simulink library "powerlib_extras"  (Simulink 6.0)
settings: Solver=ode45  SolverMode=SingleTasking  StartTime=0.0  StopTime=10.0  RelTol=1e-3
values from neighbouring files (symbols this model uses):
  Ts = get(handles.edit1,'string')    [powergui.m]
undefined symbols (not defined in the file or in its folder): Ac, Bc, Cc, Dc, Delay_discrete, dend, DiscIntNeverNeededParam, extra_sc, j, numd, test_alpha
libraries: powerlib2 x112, powerlib_extras x70, simulink_extras x25, simulink x12, powerlib_models x8
(part 9 of 9)

== system powerlib_extras/Discrete  Control Blocks/Discrete Synchronized 12-Pulse Generator/12 Flip-Flops/6 Flip-Flop1 ==
  S : Inport  Port=1  LatchInput=off
  R : Inport  Port=2  LatchInput=off
  Demux : Demux  Outputs=6
  Demux1 : Demux  Outputs=6
  Mux : Mux  Inputs=6
  S-R Flip-Flop1 : Subsystem  mask(SRFlipFlop){initial_condition=0, Ts=Ts}
      mask prompts: initial_condition "Initial condition:"; Ts "Sample time:"
      mask help: S-R Flip Flop Block
  S-R Flip-Flop2 : Subsystem  mask(SRFlipFlop){initial_condition=0, Ts=Ts}
      mask prompts: initial_condition "Initial condition:"; Ts "Sample time:"
      mask help: S-R Flip Flop Block
  S-R Flip-Flop3 : Subsystem  mask(SRFlipFlop){initial_condition=0, Ts=Ts}
      mask prompts: initial_condition "Initial condition:"; Ts "Sample time:"
      mask help: S-R Flip Flop Block
  S-R Flip-Flop4 : Subsystem  mask(SRFlipFlop){initial_condition=0, Ts=Ts}
      mask prompts: initial_condition "Initial condition:"; Ts "Sample time:"
      mask help: S-R Flip Flop Block
  S-R Flip-Flop5 : Subsystem  mask(SRFlipFlop){initial_condition=0, Ts=Ts}
      mask prompts: initial_condition "Initial condition:"; Ts "Sample time:"
      mask help: S-R Flip Flop Block
  S-R Flip-Flop6 : Subsystem  mask(SRFlipFlop){initial_condition=0, Ts=Ts}
      mask prompts: initial_condition "Initial condition:"; Ts "Sample time:"
      mask help: S-R Flip Flop Block
  Terminator{,1..5} (6 alike) : Terminator
  Q : Outport
  wires:
  Demux1/6 -> S-R Flip-Flop6/2(R)
  Demux1/5 -> S-R Flip-Flop5/2(R)
  Demux1/4 -> S-R Flip-Flop4/2(R)
  Demux1/3 -> S-R Flip-Flop3/2(R)
  Demux1/2 -> S-R Flip-Flop2/2(R)
  Demux1/1 -> S-R Flip-Flop1/2(R)
  R/1 -> Demux1/1
  Demux/5 -> S-R Flip-Flop5/1(S)
  Demux/6 -> S-R Flip-Flop6/1(S)
  S/1 -> Demux/1
  Demux/4 -> S-R Flip-Flop4/1(S)
  Demux/3 -> S-R Flip-Flop3/1(S)
  Demux/2 -> S-R Flip-Flop2/1(S)
  Demux/1 -> S-R Flip-Flop1/1(S)
  S-R Flip-Flop1/2(!Q) -> Terminator/1
  S-R Flip-Flop6/1(Q) -> Mux/6
  Mux/1 -> Q/1
  S-R Flip-Flop5/1(Q) -> Mux/5
  S-R Flip-Flop4/1(Q) -> Mux/4
  S-R Flip-Flop3/1(Q) -> Mux/3
  S-R Flip-Flop2/1(Q) -> Mux/2
  S-R Flip-Flop1/1(Q) -> Mux/1
  S-R Flip-Flop2/2(!Q) -> Terminator1/1
  S-R Flip-Flop3/2(!Q) -> Terminator2/1
  S-R Flip-Flop4/2(!Q) -> Terminator3/1
  S-R Flip-Flop5/2(!Q) -> Terminator4/1
  S-R Flip-Flop6/2(!Q) -> Terminator5/1

== system powerlib_extras/Discrete  Control Blocks/Discrete Synchronized 6-Pulse Generator/6 Flip-Flop/S-R Flip-Flop1 ==
  S : Inport  Port=1  LatchInput=off
  R : Inport  Port=2  LatchInput=off
  Demux : Demux  Outputs=2
  Logic : CombinatorialLogic  TruthTable=[0 1;0 1;1 0;0 1;1 0;0 1;1 0;1 0]
  Mux : Mux  Inputs=3
  Unit Delay : UnitDelay  Orientation=left  X0=initial_condition  SampleTime=Ts
  Q : Outport  InitialOutput=0
  !Q : Outport  Port=2  InitialOutput=1
  wires:
  Mux/1 -> Logic/1
  Logic/1 -> Demux/1
  Demux/2 -> !Q/1
  Demux/1 -> Q/1, Unit Delay/1
  Unit Delay/1 -> Mux/1
  S/1 -> Mux/2
  R/1 -> Mux/3

== system powerlib_extras/Discrete  Control Blocks/Discrete Synchronized 6-Pulse Generator/6 Flip-Flop/S-R Flip-Flop2 ==
  S : Inport  Port=1  LatchInput=off
  R : Inport  Port=2  LatchInput=off
  Demux : Demux  Outputs=2
  Logic : CombinatorialLogic  TruthTable=[0 1;0 1;1 0;0 1;1 0;0 1;1 0;1 0]
  Mux : Mux  Inputs=3
  Unit Delay : UnitDelay  Orientation=left  X0=initial_condition  SampleTime=Ts
  Q : Outport  InitialOutput=0
  !Q : Outport  Port=2  InitialOutput=1
  wires:
  R/1 -> Mux/3
  S/1 -> Mux/2
  Unit Delay/1 -> Mux/1
  Demux/1 -> Unit Delay/1, Q/1
  Demux/2 -> !Q/1
  Logic/1 -> Demux/1
  Mux/1 -> Logic/1

== system powerlib_extras/Discrete  Control Blocks/Discrete Synchronized 6-Pulse Generator/6 Flip-Flop/S-R Flip-Flop3 ==
  S : Inport  Port=1  LatchInput=off
  R : Inport  Port=2  LatchInput=off
  Demux : Demux  Outputs=2
  Logic : CombinatorialLogic  TruthTable=[0 1;0 1;1 0;0 1;1 0;0 1;1 0;1 0]
  Mux : Mux  Inputs=3
  Unit Delay : UnitDelay  Orientation=left  X0=initial_condition  SampleTime=Ts
  Q : Outport  InitialOutput=0
  !Q : Outport  Port=2  InitialOutput=1
  wires:
  Mux/1 -> Logic/1
  Logic/1 -> Demux/1
  Demux/2 -> !Q/1
  Demux/1 -> Q/1, Unit Delay/1
  Unit Delay/1 -> Mux/1
  S/1 -> Mux/2
  R/1 -> Mux/3

== system powerlib_extras/Discrete  Control Blocks/Discrete Synchronized 6-Pulse Generator/6 Flip-Flop/S-R Flip-Flop4 ==
  S : Inport  Port=1  LatchInput=off
  R : Inport  Port=2  LatchInput=off
  Demux : Demux  Outputs=2
  Logic : CombinatorialLogic  TruthTable=[0 1;0 1;1 0;0 1;1 0;0 1;1 0;1 0]
  Mux : Mux  Inputs=3
  Unit Delay : UnitDelay  Orientation=left  X0=initial_condition  SampleTime=Ts
  Q : Outport  InitialOutput=0
  !Q : Outport  Port=2  InitialOutput=1
  wires:
  R/1 -> Mux/3
  S/1 -> Mux/2
  Unit Delay/1 -> Mux/1
  Demux/1 -> Unit Delay/1, Q/1
  Demux/2 -> !Q/1
  Logic/1 -> Demux/1
  Mux/1 -> Logic/1

== system powerlib_extras/Discrete  Control Blocks/Discrete Synchronized 6-Pulse Generator/6 Flip-Flop/S-R Flip-Flop5 ==
  S : Inport  Port=1  LatchInput=off
  R : Inport  Port=2  LatchInput=off
  Demux : Demux  Outputs=2
  Logic : CombinatorialLogic  TruthTable=[0 1;0 1;1 0;0 1;1 0;0 1;1 0;1 0]
  Mux : Mux  Inputs=3
  Unit Delay : UnitDelay  Orientation=left  X0=initial_condition  SampleTime=Ts
  Q : Outport  InitialOutput=0
  !Q : Outport  Port=2  InitialOutput=1
  wires:
  Mux/1 -> Logic/1
  Logic/1 -> Demux/1
  Demux/2 -> !Q/1
  Demux/1 -> Q/1, Unit Delay/1
  Unit Delay/1 -> Mux/1
  S/1 -> Mux/2
  R/1 -> Mux/3

== system powerlib_extras/Discrete  Control Blocks/Discrete Synchronized 6-Pulse Generator/6 Flip-Flop/S-R Flip-Flop6 ==
  S : Inport  Port=1  LatchInput=off
  R : Inport  Port=2  LatchInput=off
  Demux : Demux  Outputs=2
  Logic : CombinatorialLogic  TruthTable=[0 1;0 1;1 0;0 1;1 0;0 1;1 0;1 0]
  Mux : Mux  Inputs=3
  Unit Delay : UnitDelay  Orientation=left  X0=initial_condition  SampleTime=Ts
  Q : Outport  InitialOutput=0
  !Q : Outport  Port=2  InitialOutput=1
  wires:
  R/1 -> Mux/3
  S/1 -> Mux/2
  Unit Delay/1 -> Mux/1
  Demux/1 -> Unit Delay/1, Q/1
  Demux/2 -> !Q/1
  Logic/1 -> Demux/1
  Mux/1 -> Logic/1

== system powerlib_extras/Discrete  Control Blocks/Discrete 12-Pulse HVDC Control /Functions (Discrete)/Current Regulator/Kp Linearisation ==
  note: Kp Linearization
  note: Silvano Casoria
      | Laboratoire simulation de reseaux, IREQ
  Alpha_lin : Inport  Port=1  LatchInput=off
  Kp : Inport  Port=2  LatchInput=off
  Inv : Inport  Port=3  LatchInput=off
  Min_lin : Inport  Port=4  LatchInput=off
  Max_lin : Inport  Port=5  LatchInput=off
  Constant3 : Constant  Value=On_lin
  Data Type  Conversion : DataTypeConversion  OutDataTypeMode=boolean  SaturateOnIntegerOverflow=on  RndMeth=Zero
  Logical Operator : Logic  Operator=NOT
  Logical Operator1 : Logic  Operator=NOT
  Math Function : Math  Operator=reciprocal  SaturateOnIntegerOverflow=on
  Prod2 : Product  Inputs=3  SaturateOnIntegerOverflow=on  InputSameDT=on
  S6 : Subsystem
      mask Type: Limiter with External Limits
      mask Display: disp('      Limiter\n')
  Switch : Switch  Threshold=0.5  SaturateOnIntegerOverflow=on  InputSameDT=on
  Switch1 : Switch  Threshold=0.5  SaturateOnIntegerOverflow=on  InputSameDT=on
  Trigonometric Function : Trigonometry
  Trigonometric Function1 : Trigonometry
  k : Gain  Gain=pi/180  SaturateOnIntegerOverflow=on
  k1 : Gain  Gain=pi/180  SaturateOnIntegerOverflow=on
  Kp_lin : Outport  InitialOutput=0
  wires:
  Logical Operator1/1 -> Switch1/2  "Off"
  Prod2/1 -> Switch1/3
  Switch1/1 -> Kp_lin/1
  Switch/1 -> k1/1
  k1/1 -> Trigonometric Function/1
  S6/1("  ") -> k/1
  Trigonometric Function/1 -> Prod2/1
  Logical Operator/1 -> Switch/2
  Inv/1 -> Logical Operator/1
  Kp/1 -> Switch1/1, Prod2/3
  k/1 -> Trigonometric Function1/1
  Trigonometric Function1/1 -> Math Function/1
  Math Function/1 -> Prod2/2
  Alpha_lin/1 -> S6/2(In)
  Max_lin/1 -> Switch/3, S6/1(MAX)
  Min_lin/1 -> Switch/1, S6/3(MIN)
  Constant3/1 -> Data Type  Conversion/1
  Data Type  Conversion/1 -> Logical Operator1/1

== system powerlib_extras/Discrete  Control Blocks/Discrete 12-Pulse HVDC Control /Functions (Discrete)/Current Regulator/S16 ==
  note: Gain * dt
  note: INTEGRATOR with External limits & Reset & Hold
  Max : Inport  Port=1  LatchInput=off
  Min : Inport  Port=2  LatchInput=off
  In : Inport  Port=3  LatchInput=off
  Reset : Inport  Port=4  LatchInput=off
  Hold : Inport  Port=5  LatchInput=off
  Reset Value : Inport  Port=6  LatchInput=off
  Gain1 : Gain  Gain=k*st  SaturateOnIntegerOverflow=on
  IC = ic : UnitDelay  X0=ic  SampleTime=st
  Logical Operator4 : Logic  Operator=OR
  MinMax : MinMax  Inputs=2  SaturateOnIntegerOverflow=on  InputSameDT=on
  MinMax1 : MinMax  Function=max  Inputs=2  SaturateOnIntegerOverflow=on  InputSameDT=on
  S6 : Subsystem
      mask Type: Limiter with External Limits
      mask Display: disp('      Limiter\n')
  Sum : Sum  SaturateOnIntegerOverflow=on  InputSameDT=on
  Switch2 : Switch  Threshold=0.5  SaturateOnIntegerOverflow=on  InputSameDT=on
  Switch3 : Switch  Threshold=0.5  SaturateOnIntegerOverflow=on  InputSameDT=on
  Switch7 : Switch  Threshold=0.5  SaturateOnIntegerOverflow=on  InputSameDT=on
  Out : Outport  InitialOutput=0
  wires:
  Switch7/1 -> Switch3/1, Sum/2, Switch2/1
  IC = ic/1 -> Switch7/3
  Min/1 -> MinMax1/2, Switch3/3
  Switch3/1 -> MinMax1/1
  MinMax1/1 -> S6/3(MIN)
  MinMax/1 -> S6/1(MAX)
  Reset Value/1 -> Switch7/1
  Max/1 -> MinMax/2, Switch2/3
  Switch2/1 -> MinMax/1
  Logical Operator4/1 -> Switch3/2, Switch2/2
  Reset/1 -> Logical Operator4/2, Switch7/2
  Hold/1 -> Logical Operator4/1
  S6/1("  ") -> IC = ic/1, Out/1
  Sum/1 -> S6/2(In)
  In/1 -> Gain1/1
  Gain1/1 -> Sum/1

== system powerlib_extras/Discrete  Control Blocks/Discrete 12-Pulse HVDC Control /Functions (Discrete)/Current Regulator/S6 ==
  note: Limiter
      | with external
      | limits
  MAX : Inport  Port=1  LatchInput=off
  In : Inport  Port=2  LatchInput=off
  MIN : Inport  Port=3  LatchInput=off
  MinMax : MinMax  Function=max  Inputs=2  SaturateOnIntegerOverflow=on  InputSameDT=on
  MinMax1 : MinMax  Inputs=2  SaturateOnIntegerOverflow=on  InputSameDT=on
  "  " : Outport  InitialOutput=0
  wires:
  MinMax1/1 -> MinMax/2
  MAX/1 -> MinMax1/1
  MIN/1 -> MinMax/1
  MinMax/1 -> "  "/1
  In/1 -> MinMax1/2

== system powerlib_extras/Discrete  Control Blocks/Discrete 12-Pulse HVDC Control /Functions (Discrete)/VDCOL/PB_R ==
  note: LOW PASS Filter & RESET
      | (Zoh methode)
  note: Silvano Casoria
      | Laboratoire simulation de reseaux, IREQ
  "In " : Inport  Port=1  LatchInput=off
  Reset : Inport  Port=2  LatchInput=off
  T : Inport  Port=3  LatchInput=off
  Constant : Constant  Value=dt
  IC= ic : UnitDelay  Orientation=left  X0=ic  SampleTime=dt
  Math Function : Math  Operator=reciprocal  SaturateOnIntegerOverflow=on
  Product : Product  Inputs=3  SaturateOnIntegerOverflow=on  InputSameDT=on
  Sum : Sum  Inputs=+-  SaturateOnIntegerOverflow=on  InputSameDT=on
  Sum1 : Sum  SaturateOnIntegerOverflow=on  InputSameDT=on
  Switch : Switch  Threshold=0.5  SaturateOnIntegerOverflow=on  InputSameDT=on
  Out : Outport  InitialOutput=0
  wires:
  Constant/1 -> Product/3
  T/1 -> Math Function/1
  Math Function/1 -> Product/1
  Sum/1 -> Product/2
  Product/1 -> Sum1/1
  Switch/1 -> IC= ic/1
  Sum1/1 -> Switch/3, Out/1
  Reset/1 -> Switch/2
  "In "/1 -> Switch/1, Sum/1
  IC= ic/1 -> Sum1/2, Sum/2

== system powerlib_extras/Discrete  Control Blocks/Discrete 12-Pulse HVDC Control /Functions (Discrete)/Voltage Regulator/Kp Linearisation ==
  note: Kp Linearization
  Alpha_lin : Inport  Port=1  LatchInput=off
  Kp : Inport  Port=2  LatchInput=off
  Inv : Inport  Port=3  LatchInput=off
  Min_lin : Inport  Port=4  LatchInput=off
  Max_lin : Inport  Port=5  LatchInput=off
  Constant3 : Constant  Value=On_lin
  Data Type  Conversion : DataTypeConversion  OutDataTypeMode=boolean  SaturateOnIntegerOverflow=on  RndMeth=Zero
  Logical Operator : Logic  Operator=NOT
  Logical Operator1 : Logic  Operator=NOT
  Math Function : Math  Operator=reciprocal  SaturateOnIntegerOverflow=on
  Prod2 : Product  Inputs=3  SaturateOnIntegerOverflow=on  InputSameDT=on
  S6 : Subsystem
      mask Type: Limiter with External Limits
      mask Display: disp('      Limiter\n')
  Switch : Switch  Threshold=0.5  SaturateOnIntegerOverflow=on  InputSameDT=on
  Switch1 : Switch  Threshold=0.5  SaturateOnIntegerOverflow=on  InputSameDT=on
  Trigonometric Function : Trigonometry
  Trigonometric Function1 : Trigonometry
  k : Gain  Gain=pi/180  SaturateOnIntegerOverflow=on
  k1 : Gain  Gain=pi/180  SaturateOnIntegerOverflow=on
  Kp_lin : Outport  InitialOutput=0
  wires:
  Min_lin/1 -> S6/3(MIN), Switch/1
  Max_lin/1 -> S6/1(MAX), Switch/3
  Alpha_lin/1 -> S6/2(In)
  Math Function/1 -> Prod2/2
  Trigonometric Function1/1 -> Math Function/1
  k/1 -> Trigonometric Function1/1
  Kp/1 -> Prod2/3, Switch1/1
  Inv/1 -> Logical Operator/1
  Logical Operator/1 -> Switch/2
  Trigonometric Function/1 -> Prod2/1
  S6/1("  ") -> k/1
  k1/1 -> Trigonometric Function/1
  Switch/1 -> k1/1
  Switch1/1 -> Kp_lin/1
  Prod2/1 -> Switch1/3
  Logical Operator1/1 -> Switch1/2  "Off"
  Constant3/1 -> Data Type  Conversion/1
  Data Type  Conversion/1 -> Logical Operator1/1

== system powerlib_extras/Discrete  Control Blocks/Discrete 12-Pulse HVDC Control /Functions (Discrete)/Voltage Regulator/S16 ==
  note: INTEGRATOR with External limits & Reset & Hold
  note: Gain * dt
  Max : Inport  Port=1  LatchInput=off
  Min : Inport  Port=2  LatchInput=off
  In : Inport  Port=3  LatchInput=off
  Reset : Inport  Port=4  LatchInput=off
  Hold : Inport  Port=5  LatchInput=off
  Reset Value : Inport  Port=6  LatchInput=off
  Gain1 : Gain  Gain=k*st  SaturateOnIntegerOverflow=on
  IC = ic : UnitDelay  X0=ic  SampleTime=st
  Logical Operator4 : Logic  Operator=OR
  MinMax : MinMax  Inputs=2  SaturateOnIntegerOverflow=on  InputSameDT=on
  MinMax1 : MinMax  Function=max  Inputs=2  SaturateOnIntegerOverflow=on  InputSameDT=on
  S6 : Subsystem
      mask Type: Limiter with External Limits
      mask Display: disp('      Limiter\n')
  Sum : Sum  SaturateOnIntegerOverflow=on  InputSameDT=on
  Switch2 : Switch  Threshold=0.5  SaturateOnIntegerOverflow=on  InputSameDT=on
  Switch3 : Switch  Threshold=0.5  SaturateOnIntegerOverflow=on  InputSameDT=on
  Switch7 : Switch  Threshold=0.5  SaturateOnIntegerOverflow=on  InputSameDT=on
  Out : Outport  InitialOutput=0
  wires:
  Gain1/1 -> Sum/1
  In/1 -> Gain1/1
  Sum/1 -> S6/2(In)
  S6/1("  ") -> Out/1, IC = ic/1
  Hold/1 -> Logical Operator4/1
  Reset/1 -> Switch7/2, Logical Operator4/2
  Logical Operator4/1 -> Switch2/2, Switch3/2
  Switch2/1 -> MinMax/1
  Max/1 -> Switch2/3, MinMax/2
  Reset Value/1 -> Switch7/1
  MinMax/1 -> S6/1(MAX)
  MinMax1/1 -> S6/3(MIN)
  Switch3/1 -> MinMax1/1
  Min/1 -> Switch3/3, MinMax1/2
  IC = ic/1 -> Switch7/3
  Switch7/1 -> Switch2/1, Sum/2, Switch3/1

== system powerlib_extras/Discrete  Control Blocks/Discrete 12-Pulse HVDC Control /Functions (Discrete)/Voltage Regulator/S6 ==
  note: Limiter
      | with external
      | limits
  MAX : Inport  Port=1  LatchInput=off
  In : Inport  Port=2  LatchInput=off
  MIN : Inport  Port=3  LatchInput=off
  MinMax : MinMax  Function=max  Inputs=2  SaturateOnIntegerOverflow=on  InputSameDT=on
  MinMax1 : MinMax  Inputs=2  SaturateOnIntegerOverflow=on  InputSameDT=on
  "  " : Outport  InitialOutput=0
  wires:
  In/1 -> MinMax1/2
  MinMax/1 -> "  "/1
  MIN/1 -> MinMax/1
  MAX/1 -> MinMax1/1
  MinMax1/1 -> MinMax/2

== system powerlib_extras/Discrete  Control Blocks/Discrete HVDC Controller/Current Regulator/Kp Linearisation/S6 ==
  note: Limiter
      | with external
      | limits
  MAX : Inport  Port=1  LatchInput=off
  In : Inport  Port=2  LatchInput=off
  MIN : Inport  Port=3  LatchInput=off
  MinMax : MinMax  Function=max  Inputs=2  SaturateOnIntegerOverflow=on  InputSameDT=on
  MinMax1 : MinMax  Inputs=2  SaturateOnIntegerOverflow=on  InputSameDT=on
  "  " : Outport  InitialOutput=0
  wires:
  MinMax1/1 -> MinMax/2
  MAX/1 -> MinMax1/1
  MIN/1 -> MinMax/1
  MinMax/1 -> "  "/1
  In/1 -> MinMax1/2

== system powerlib_extras/Discrete  Control Blocks/Discrete HVDC Controller/Current Regulator/S16/S6 ==
  note: Limiter
      | with external
      | limits
  MAX : Inport  Port=1  LatchInput=off
  In : Inport  Port=2  LatchInput=off
  MIN : Inport  Port=3  LatchInput=off
  MinMax : MinMax  Function=max  Inputs=2  SaturateOnIntegerOverflow=on  InputSameDT=on
  MinMax1 : MinMax  Inputs=2  SaturateOnIntegerOverflow=on  InputSameDT=on
  "  " : Outport  InitialOutput=0
  wires:
  MinMax1/1 -> MinMax/2
  MAX/1 -> MinMax1/1
  MIN/1 -> MinMax/1
  MinMax/1 -> "  "/1
  In/1 -> MinMax1/2

== system powerlib_extras/Discrete  Control Blocks/Discrete HVDC Controller/Gamma Regulator/Gamma Regulator/Kp Linearisation ==
  note: Kp Linearization
  Alpha_lin : Inport  Port=1  LatchInput=off
  Kp : Inport  Port=2  LatchInput=off
  Inv : Inport  Port=3  LatchInput=off
  Min_lin : Inport  Port=4  LatchInput=off
  Max_lin : Inport  Port=5  LatchInput=off
  Constant3 : Constant  Value=On_lin
  Data Type  Conversion : DataTypeConversion  OutDataTypeMode=boolean  SaturateOnIntegerOverflow=on  RndMeth=Zero
  Logical Operator : Logic  Operator=NOT
  Logical Operator1 : Logic  Operator=NOT
  Math Function : Math  Operator=reciprocal  SaturateOnIntegerOverflow=on
  Prod2 : Product  Inputs=3  SaturateOnIntegerOverflow=on  InputSameDT=on
  S6 : Subsystem
      mask Type: Limiter with External Limits
      mask Display: disp('      Limiter\n')
  Switch : Switch  Threshold=0.5  SaturateOnIntegerOverflow=on  InputSameDT=on
  Switch1 : Switch  Threshold=0.5  SaturateOnIntegerOverflow=on  InputSameDT=on
  Trigonometric Function : Trigonometry
  Trigonometric Function1 : Trigonometry
  k : Gain  Gain=pi/180  SaturateOnIntegerOverflow=on
  k1 : Gain  Gain=pi/180  SaturateOnIntegerOverflow=on
  Kp_lin : Outport  InitialOutput=0
  wires:
  Data Type  Conversion/1 -> Logical Operator1/1
  Constant3/1 -> Data Type  Conversion/1
  Logical Operator1/1 -> Switch1/2  "Off"
  Prod2/1 -> Switch1/3
  Switch1/1 -> Kp_lin/1
  Switch/1 -> k1/1
  k1/1 -> Trigonometric Function/1
  S6/1("  ") -> k/1
  Trigonometric Function/1 -> Prod2/1
  Logical Operator/1 -> Switch/2
  Inv/1 -> Logical Operator/1
  Kp/1 -> Switch1/1, Prod2/3
  k/1 -> Trigonometric Function1/1
  Trigonometric Function1/1 -> Math Function/1
  Math Function/1 -> Prod2/2
  Alpha_lin/1 -> S6/2(In)
  Max_lin/1 -> Switch/3, S6/1(MAX)
  Min_lin/1 -> Switch/1, S6/3(MIN)

== system powerlib_extras/Discrete  Control Blocks/Discrete HVDC Controller/Gamma Regulator/Gamma Regulator/S16 ==
  note: Gain * dt
  note: INTEGRATOR with External limits & Reset & Hold
  Max : Inport  Port=1  LatchInput=off
  Min : Inport  Port=2  LatchInput=off
  In : Inport  Port=3  LatchInput=off
  Reset : Inport  Port=4  LatchInput=off
  Hold : Inport  Port=5  LatchInput=off
  Reset Value : Inport  Port=6  LatchInput=off
  Gain1 : Gain  Gain=k*st  SaturateOnIntegerOverflow=on
  IC = ic : UnitDelay  X0=ic  SampleTime=st
  Logical Operator4 : Logic  Operator=OR
  MinMax : MinMax  Inputs=2  SaturateOnIntegerOverflow=on  InputSameDT=on
  MinMax1 : MinMax  Function=max  Inputs=2  SaturateOnIntegerOverflow=on  InputSameDT=on
  S6 : Subsystem
      mask Type: Limiter with External Limits
      mask Display: disp('      Limiter\n')
  Sum : Sum  SaturateOnIntegerOverflow=on  InputSameDT=on
  Switch2 : Switch  Threshold=0.5  SaturateOnIntegerOverflow=on  InputSameDT=on
  Switch3 : Switch  Threshold=0.5  SaturateOnIntegerOverflow=on  InputSameDT=on
  Switch7 : Switch  Threshold=0.5  SaturateOnIntegerOverflow=on  InputSameDT=on
  Out : Outport  InitialOutput=0
  wires:
  Switch7/1 -> Switch3/1, Sum/2, Switch2/1
  IC = ic/1 -> Switch7/3
  Min/1 -> MinMax1/2, Switch3/3
  Switch3/1 -> MinMax1/1
  MinMax1/1 -> S6/3(MIN)
  MinMax/1 -> S6/1(MAX)
  Reset Value/1 -> Switch7/1
  Max/1 -> MinMax/2, Switch2/3
  Switch2/1 -> MinMax/1
  Logical Operator4/1 -> Switch3/2, Switch2/2
  Reset/1 -> Logical Operator4/2, Switch7/2
  Hold/1 -> Logical Operator4/1
  S6/1("  ") -> IC = ic/1, Out/1
  Sum/1 -> S6/2(In)
  In/1 -> Gain1/1
  Gain1/1 -> Sum/1

== system powerlib_extras/Discrete  Control Blocks/Discrete HVDC Controller/Gamma Regulator/Gamma Regulator/S6 ==
  note: Limiter
      | with external
      | limits
  MAX : Inport  Port=1  LatchInput=off
  In : Inport  Port=2  LatchInput=off
  MIN : Inport  Port=3  LatchInput=off
  MinMax : MinMax  Function=max  Inputs=2  SaturateOnIntegerOverflow=on  InputSameDT=on
  MinMax1 : MinMax  Inputs=2  SaturateOnIntegerOverflow=on  InputSameDT=on
  "  " : Outport  InitialOutput=0
  wires:
  MinMax1/1 -> MinMax/2
  MAX/1 -> MinMax1/1
  MIN/1 -> MinMax/1
  MinMax/1 -> "  "/1
  In/1 -> MinMax1/2

== system powerlib_extras/Discrete  Control Blocks/Discrete HVDC Controller/Voltage Regulator/Voltage Regulator/Kp Linearisation ==
  note: Kp Linearization
  Alpha_lin : Inport  Port=1  LatchInput=off
  Kp : Inport  Port=2  LatchInput=off
  Inv : Inport  Port=3  LatchInput=off
  Min_lin : Inport  Port=4  LatchInput=off
  Max_lin : Inport  Port=5  LatchInput=off
  Constant3 : Constant  Value=On_lin
  Data Type  Conversion : DataTypeConversion  OutDataTypeMode=boolean  SaturateOnIntegerOverflow=on  RndMeth=Zero
  Logical Operator : Logic  Operator=NOT
  Logical Operator1 : Logic  Operator=NOT
  Math Function : Math  Operator=reciprocal  SaturateOnIntegerOverflow=on
  Prod2 : Product  Inputs=3  SaturateOnIntegerOverflow=on  InputSameDT=on
  S6 : Subsystem
      mask Type: Limiter with External Limits
      mask Display: disp('      Limiter\n')
  Switch : Switch  Threshold=0.5  SaturateOnIntegerOverflow=on  InputSameDT=on
  Switch1 : Switch  Threshold=0.5  SaturateOnIntegerOverflow=on  InputSameDT=on
  Trigonometric Function : Trigonometry
  Trigonometric Function1 : Trigonometry
  k : Gain  Gain=pi/180  SaturateOnIntegerOverflow=on
  k1 : Gain  Gain=pi/180  SaturateOnIntegerOverflow=on
  Kp_lin : Outport  InitialOutput=0
  wires:
  Min_lin/1 -> S6/3(MIN), Switch/1
  Max_lin/1 -> S6/1(MAX), Switch/3
  Alpha_lin/1 -> S6/2(In)
  Math Function/1 -> Prod2/2
  Trigonometric Function1/1 -> Math Function/1
  k/1 -> Trigonometric Function1/1
  Kp/1 -> Prod2/3, Switch1/1
  Inv/1 -> Logical Operator/1
  Logical Operator/1 -> Switch/2
  Trigonometric Function/1 -> Prod2/1
  S6/1("  ") -> k/1
  k1/1 -> Trigonometric Function/1
  Switch/1 -> k1/1
  Switch1/1 -> Kp_lin/1
  Prod2/1 -> Switch1/3
  Logical Operator1/1 -> Switch1/2  "Off"
  Constant3/1 -> Data Type  Conversion/1
  Data Type  Conversion/1 -> Logical Operator1/1

== system powerlib_extras/Discrete  Control Blocks/Discrete HVDC Controller/Voltage Regulator/Voltage Regulator/S16 ==
  note: INTEGRATOR with External limits & Reset & Hold
  note: Gain * dt
  Max : Inport  Port=1  LatchInput=off
  Min : Inport  Port=2  LatchInput=off
  In : Inport  Port=3  LatchInput=off
  Reset : Inport  Port=4  LatchInput=off
  Hold : Inport  Port=5  LatchInput=off
  Reset Value : Inport  Port=6  LatchInput=off
  Gain1 : Gain  Gain=k*st  SaturateOnIntegerOverflow=on
  IC = ic : UnitDelay  X0=ic  SampleTime=st
  Logical Operator4 : Logic  Operator=OR
  MinMax : MinMax  Inputs=2  SaturateOnIntegerOverflow=on  InputSameDT=on
  MinMax1 : MinMax  Function=max  Inputs=2  SaturateOnIntegerOverflow=on  InputSameDT=on
  S6 : Subsystem
      mask Type: Limiter with External Limits
      mask Display: disp('      Limiter\n')
  Sum : Sum  SaturateOnIntegerOverflow=on  InputSameDT=on
  Switch2 : Switch  Threshold=0.5  SaturateOnIntegerOverflow=on  InputSameDT=on
  Switch3 : Switch  Threshold=0.5  SaturateOnIntegerOverflow=on  InputSameDT=on
  Switch7 : Switch  Threshold=0.5  SaturateOnIntegerOverflow=on  InputSameDT=on
  Out : Outport  InitialOutput=0
  wires:
  Gain1/1 -> Sum/1
  In/1 -> Gain1/1
  Sum/1 -> S6/2(In)
  S6/1("  ") -> Out/1, IC = ic/1
  Hold/1 -> Logical Operator4/1
  Reset/1 -> Switch7/2, Logical Operator4/2
  Logical Operator4/1 -> Switch2/2, Switch3/2
  Switch2/1 -> MinMax/1
  Max/1 -> Switch2/3, MinMax/2
  Reset Value/1 -> Switch7/1
  MinMax/1 -> S6/1(MAX)
  MinMax1/1 -> S6/3(MIN)
  Switch3/1 -> MinMax1/1
  Min/1 -> Switch3/3, MinMax1/2
  IC = ic/1 -> Switch7/3
  Switch7/1 -> Switch2/1, Sum/2, Switch3/1

== system powerlib_extras/Discrete  Control Blocks/Discrete HVDC Controller/Voltage Regulator/Voltage Regulator/S6 ==
  note: Limiter
      | with external
      | limits
  MAX : Inport  Port=1  LatchInput=off
  In : Inport  Port=2  LatchInput=off
  MIN : Inport  Port=3  LatchInput=off
  MinMax : MinMax  Function=max  Inputs=2  SaturateOnIntegerOverflow=on  InputSameDT=on
  MinMax1 : MinMax  Inputs=2  SaturateOnIntegerOverflow=on  InputSameDT=on
  "  " : Outport  InitialOutput=0
  wires:
  In/1 -> MinMax1/2
  MinMax/1 -> "  "/1
  MIN/1 -> MinMax/1
  MAX/1 -> MinMax1/1
  MinMax1/1 -> MinMax/2

== system powerlib_extras/Discrete  Control Blocks/Discrete SV PWM Generator/SV Modulator Pattern #1/Generate  pulse pattern/Determine interval of the PWM period based on Ta Tb and To ==
  TaTbTo : Inport  Port=1  LatchInput=off
  Constant7 : Constant
  Demux1 : Demux  Outputs=6
  Relational Operator{,1..5} (6 alike) : RelationalOperator
  Subsystem : Subsystem
  Sum1 : Sum  Inputs=+++++++  SaturateOnIntegerOverflow=on
  Triangle : simulink/Sources/Repeating Sequence  rep_seq_t=[0 1/Fc]  rep_seq_y=[0 1/Fc]
  Tn : Outport
  wires:
  TaTbTo/1 -> Subsystem/1(TaTbTo)
  Subsystem/1(Timing) -> Demux1/1
  Triangle/1 -> Relational Operator4/1, Relational Operator3/1, Relational Operator2/1, Relational Operator1/1, Relational Operator/1, Relational Operator5/1
  Relational Operator4/1 -> Sum1/7
  Relational Operator3/1 -> Sum1/6
  Relational Operator2/1 -> Sum1/5
  Relational Operator1/1 -> Sum1/4
  Relational Operator/1 -> Sum1/3
  Relational Operator5/1 -> Sum1/2
  Constant7/1 -> Sum1/1
  Demux1/1 -> Relational Operator5/2
  Demux1/2 -> Relational Operator/2
  Demux1/3 -> Relational Operator1/2
  Demux1/4 -> Relational Operator2/2
  Demux1/5 -> Relational Operator3/2
  Demux1/6 -> Relational Operator4/2
  Sum1/1 -> Tn/1

== system powerlib_extras/Discrete  Control Blocks/Discrete Synchronized 12-Pulse Generator/12 Flip-Flops/6 Flip-Flop/S-R Flip-Flop1 ==
  S : Inport  Port=1  LatchInput=off
  R : Inport  Port=2  LatchInput=off
  Demux : Demux  Outputs=2
  Logic : CombinatorialLogic  TruthTable=[0 1;0 1;1 0;0 1;1 0;0 1;1 0;1 0]
  Mux : Mux  Inputs=3
  Unit Delay : UnitDelay  Orientation=left  X0=initial_condition  SampleTime=Ts
  Q : Outport  InitialOutput=0
  !Q : Outport  Port=2  InitialOutput=1
  wires:
  R/1 -> Mux/3
  S/1 -> Mux/2
  Unit Delay/1 -> Mux/1
  Demux/1 -> Unit Delay/1, Q/1
  Demux/2 -> !Q/1
  Logic/1 -> Demux/1
  Mux/1 -> Logic/1

== system powerlib_extras/Discrete  Control Blocks/Discrete Synchronized 12-Pulse Generator/12 Flip-Flops/6 Flip-Flop/S-R Flip-Flop2 ==
  S : Inport  Port=1  LatchInput=off
  R : Inport  Port=2  LatchInput=off
  Demux : Demux  Outputs=2
  Logic : CombinatorialLogic  TruthTable=[0 1;0 1;1 0;0 1;1 0;0 1;1 0;1 0]
  Mux : Mux  Inputs=3
  Unit Delay : UnitDelay  Orientation=left  X0=initial_condition  SampleTime=Ts
  Q : Outport  InitialOutput=0
  !Q : Outport  Port=2  InitialOutput=1
  wires:
  Mux/1 -> Logic/1
  Logic/1 -> Demux/1
  Demux/2 -> !Q/1
  Demux/1 -> Q/1, Unit Delay/1
  Unit Delay/1 -> Mux/1
  S/1 -> Mux/2
  R/1 -> Mux/3

== system powerlib_extras/Discrete  Control Blocks/Discrete Synchronized 12-Pulse Generator/12 Flip-Flops/6 Flip-Flop/S-R Flip-Flop3 ==
  S : Inport  Port=1  LatchInput=off
  R : Inport  Port=2  LatchInput=off
  Demux : Demux  Outputs=2
  Logic : CombinatorialLogic  TruthTable=[0 1;0 1;1 0;0 1;1 0;0 1;1 0;1 0]
  Mux : Mux  Inputs=3
  Unit Delay : UnitDelay  Orientation=left  X0=initial_condition  SampleTime=Ts
  Q : Outport  InitialOutput=0
  !Q : Outport  Port=2  InitialOutput=1
  wires:
  R/1 -> Mux/3
  S/1 -> Mux/2
  Unit Delay/1 -> Mux/1
  Demux/1 -> Unit Delay/1, Q/1
  Demux/2 -> !Q/1
  Logic/1 -> Demux/1
  Mux/1 -> Logic/1

== system powerlib_extras/Discrete  Control Blocks/Discrete Synchronized 12-Pulse Generator/12 Flip-Flops/6 Flip-Flop/S-R Flip-Flop4 ==
  S : Inport  Port=1  LatchInput=off
  R : Inport  Port=2  LatchInput=off
  Demux : Demux  Outputs=2
  Logic : CombinatorialLogic  TruthTable=[0 1;0 1;1 0;0 1;1 0;0 1;1 0;1 0]
  Mux : Mux  Inputs=3
  Unit Delay : UnitDelay  Orientation=left  X0=initial_condition  SampleTime=Ts
  Q : Outport  InitialOutput=0
  !Q : Outport  Port=2  InitialOutput=1
  wires:
  Mux/1 -> Logic/1
  Logic/1 -> Demux/1
  Demux/2 -> !Q/1
  Demux/1 -> Q/1, Unit Delay/1
  Unit Delay/1 -> Mux/1
  S/1 -> Mux/2
  R/1 -> Mux/3

== system powerlib_extras/Discrete  Control Blocks/Discrete Synchronized 12-Pulse Generator/12 Flip-Flops/6 Flip-Flop/S-R Flip-Flop5 ==
  S : Inport  Port=1  LatchInput=off
  R : Inport  Port=2  LatchInput=off
  Demux : Demux  Outputs=2
  Logic : CombinatorialLogic  TruthTable=[0 1;0 1;1 0;0 1;1 0;0 1;1 0;1 0]
  Mux : Mux  Inputs=3
  Unit Delay : UnitDelay  Orientation=left  X0=initial_condition  SampleTime=Ts
  Q : Outport  InitialOutput=0
  !Q : Outport  Port=2  InitialOutput=1
  wires:
  R/1 -> Mux/3
  S/1 -> Mux/2
  Unit Delay/1 -> Mux/1
  Demux/1 -> Unit Delay/1, Q/1
  Demux/2 -> !Q/1
  Logic/1 -> Demux/1
  Mux/1 -> Logic/1

== system powerlib_extras/Discrete  Control Blocks/Discrete Synchronized 12-Pulse Generator/12 Flip-Flops/6 Flip-Flop/S-R Flip-Flop6 ==
  S : Inport  Port=1  LatchInput=off
  R : Inport  Port=2  LatchInput=off
  Demux : Demux  Outputs=2
  Logic : CombinatorialLogic  TruthTable=[0 1;0 1;1 0;0 1;1 0;0 1;1 0;1 0]
  Mux : Mux  Inputs=3
  Unit Delay : UnitDelay  Orientation=left  X0=initial_condition  SampleTime=Ts
  Q : Outport  InitialOutput=0
  !Q : Outport  Port=2  InitialOutput=1
  wires:
  Mux/1 -> Logic/1
  Logic/1 -> Demux/1
  Demux/2 -> !Q/1
  Demux/1 -> Q/1, Unit Delay/1
  Unit Delay/1 -> Mux/1
  S/1 -> Mux/2
  R/1 -> Mux/3

== system powerlib_extras/Discrete  Control Blocks/Discrete Synchronized 12-Pulse Generator/12 Flip-Flops/6 Flip-Flop1/S-R Flip-Flop1 ==
  S : Inport  Port=1  LatchInput=off
  R : Inport  Port=2  LatchInput=off
  Demux : Demux  Outputs=2
  Logic : CombinatorialLogic  TruthTable=[0 1;0 1;1 0;0 1;1 0;0 1;1 0;1 0]
  Mux : Mux  Inputs=3
  Unit Delay : UnitDelay  Orientation=left  X0=initial_condition  SampleTime=Ts
  Q : Outport  InitialOutput=0
  !Q : Outport  Port=2  InitialOutput=1
  wires:
  Mux/1 -> Logic/1
  Logic/1 -> Demux/1
  Demux/2 -> !Q/1
  Demux/1 -> Q/1, Unit Delay/1
  Unit Delay/1 -> Mux/1
  S/1 -> Mux/2
  R/1 -> Mux/3

== system powerlib_extras/Discrete  Control Blocks/Discrete Synchronized 12-Pulse Generator/12 Flip-Flops/6 Flip-Flop1/S-R Flip-Flop2 ==
  S : Inport  Port=1  LatchInput=off
  R : Inport  Port=2  LatchInput=off
  Demux : Demux  Outputs=2
  Logic : CombinatorialLogic  TruthTable=[0 1;0 1;1 0;0 1;1 0;0 1;1 0;1 0]
  Mux : Mux  Inputs=3
  Unit Delay : UnitDelay  Orientation=left  X0=initial_condition  SampleTime=Ts
  Q : Outport  InitialOutput=0
  !Q : Outport  Port=2  InitialOutput=1
  wires:
  R/1 -> Mux/3
  S/1 -> Mux/2
  Unit Delay/1 -> Mux/1
  Demux/1 -> Unit Delay/1, Q/1
  Demux/2 -> !Q/1
  Logic/1 -> Demux/1
  Mux/1 -> Logic/1

== system powerlib_extras/Discrete  Control Blocks/Discrete Synchronized 12-Pulse Generator/12 Flip-Flops/6 Flip-Flop1/S-R Flip-Flop3 ==
  S : Inport  Port=1  LatchInput=off
  R : Inport  Port=2  LatchInput=off
  Demux : Demux  Outputs=2
  Logic : CombinatorialLogic  TruthTable=[0 1;0 1;1 0;0 1;1 0;0 1;1 0;1 0]
  Mux : Mux  Inputs=3
  Unit Delay : UnitDelay  Orientation=left  X0=initial_condition  SampleTime=Ts
  Q : Outport  InitialOutput=0
  !Q : Outport  Port=2  InitialOutput=1
  wires:
  Mux/1 -> Logic/1
  Logic/1 -> Demux/1
  Demux/2 -> !Q/1
  Demux/1 -> Q/1, Unit Delay/1
  Unit Delay/1 -> Mux/1
  S/1 -> Mux/2
  R/1 -> Mux/3

== system powerlib_extras/Discrete  Control Blocks/Discrete Synchronized 12-Pulse Generator/12 Flip-Flops/6 Flip-Flop1/S-R Flip-Flop4 ==
  S : Inport  Port=1  LatchInput=off
  R : Inport  Port=2  LatchInput=off
  Demux : Demux  Outputs=2
  Logic : CombinatorialLogic  TruthTable=[0 1;0 1;1 0;0 1;1 0;0 1;1 0;1 0]
  Mux : Mux  Inputs=3
  Unit Delay : UnitDelay  Orientation=left  X0=initial_condition  SampleTime=Ts
  Q : Outport  InitialOutput=0
  !Q : Outport  Port=2  InitialOutput=1
  wires:
  R/1 -> Mux/3
  S/1 -> Mux/2
  Unit Delay/1 -> Mux/1
  Demux/1 -> Unit Delay/1, Q/1
  Demux/2 -> !Q/1
  Logic/1 -> Demux/1
  Mux/1 -> Logic/1

== system powerlib_extras/Discrete  Control Blocks/Discrete Synchronized 12-Pulse Generator/12 Flip-Flops/6 Flip-Flop1/S-R Flip-Flop5 ==
  S : Inport  Port=1  LatchInput=off
  R : Inport  Port=2  LatchInput=off
  Demux : Demux  Outputs=2
  Logic : CombinatorialLogic  TruthTable=[0 1;0 1;1 0;0 1;1 0;0 1;1 0;1 0]
  Mux : Mux  Inputs=3
  Unit Delay : UnitDelay  Orientation=left  X0=initial_condition  SampleTime=Ts
  Q : Outport  InitialOutput=0
  !Q : Outport  Port=2  InitialOutput=1
  wires:
  Mux/1 -> Logic/1
  Logic/1 -> Demux/1
  Demux/2 -> !Q/1
  Demux/1 -> Q/1, Unit Delay/1
  Unit Delay/1 -> Mux/1
  S/1 -> Mux/2
  R/1 -> Mux/3

== system powerlib_extras/Discrete  Control Blocks/Discrete Synchronized 12-Pulse Generator/12 Flip-Flops/6 Flip-Flop1/S-R Flip-Flop6 ==
  S : Inport  Port=1  LatchInput=off
  R : Inport  Port=2  LatchInput=off
  Demux : Demux  Outputs=2
  Logic : CombinatorialLogic  TruthTable=[0 1;0 1;1 0;0 1;1 0;0 1;1 0;1 0]
  Mux : Mux  Inputs=3
  Unit Delay : UnitDelay  Orientation=left  X0=initial_condition  SampleTime=Ts
  Q : Outport  InitialOutput=0
  !Q : Outport  Port=2  InitialOutput=1
  wires:
  R/1 -> Mux/3
  S/1 -> Mux/2
  Unit Delay/1 -> Mux/1
  Demux/1 -> Unit Delay/1, Q/1
  Demux/2 -> !Q/1
  Logic/1 -> Demux/1
  Mux/1 -> Logic/1

== system powerlib_extras/Discrete  Control Blocks/Discrete 12-Pulse HVDC Control /Functions (Discrete)/Current Regulator/Kp Linearisation/S6 ==
  note: Limiter
      | with external
      | limits
  MAX : Inport  Port=1  LatchInput=off
  In : Inport  Port=2  LatchInput=off
  MIN : Inport  Port=3  LatchInput=off
  MinMax : MinMax  Function=max  Inputs=2  SaturateOnIntegerOverflow=on  InputSameDT=on
  MinMax1 : MinMax  Inputs=2  SaturateOnIntegerOverflow=on  InputSameDT=on
  "  " : Outport  InitialOutput=0
  wires:
  In/1 -> MinMax1/2
  MinMax/1 -> "  "/1
  MIN/1 -> MinMax/1
  MAX/1 -> MinMax1/1
  MinMax1/1 -> MinMax/2

== system powerlib_extras/Discrete  Control Blocks/Discrete 12-Pulse HVDC Control /Functions (Discrete)/Current Regulator/S16/S6 ==
  note: Silvano Casoria
      | Laboratoire simulation de reseaux, IREQ
  note: Limiter
      | with external
      | limits
  MAX : Inport  Port=1  LatchInput=off
  In : Inport  Port=2  LatchInput=off
  MIN : Inport  Port=3  LatchInput=off
  MinMax : MinMax  Function=max  Inputs=2  SaturateOnIntegerOverflow=on  InputSameDT=on
  MinMax1 : MinMax  Inputs=2  SaturateOnIntegerOverflow=on  InputSameDT=on
  "  " : Outport  InitialOutput=0
  wires:
  In/1 -> MinMax1/2
  MinMax/1 -> "  "/1
  MIN/1 -> MinMax/1
  MAX/1 -> MinMax1/1
  MinMax1/1 -> MinMax/2

== system powerlib_extras/Discrete  Control Blocks/Discrete 12-Pulse HVDC Control /Functions (Discrete)/Voltage Regulator/Kp Linearisation/S6 ==
  note: Limiter
      | with external
      | limits
  MAX : Inport  Port=1  LatchInput=off
  In : Inport  Port=2  LatchInput=off
  MIN : Inport  Port=3  LatchInput=off
  MinMax : MinMax  Function=max  Inputs=2  SaturateOnIntegerOverflow=on  InputSameDT=on
  MinMax1 : MinMax  Inputs=2  SaturateOnIntegerOverflow=on  InputSameDT=on
  "  " : Outport  InitialOutput=0
  wires:
  In/1 -> MinMax1/2
  MinMax/1 -> "  "/1
  MIN/1 -> MinMax/1
  MAX/1 -> MinMax1/1
  MinMax1/1 -> MinMax/2

== system powerlib_extras/Discrete  Control Blocks/Discrete 12-Pulse HVDC Control /Functions (Discrete)/Voltage Regulator/S16/S6 ==
  note: Limiter
      | with external
      | limits
  note: Silvano Casoria
      | Laboratoire simulation de reseaux, IREQ
  MAX : Inport  Port=1  LatchInput=off
  In : Inport  Port=2  LatchInput=off
  MIN : Inport  Port=3  LatchInput=off
  MinMax : MinMax  Function=max  Inputs=2  SaturateOnIntegerOverflow=on  InputSameDT=on
  MinMax1 : MinMax  Inputs=2  SaturateOnIntegerOverflow=on  InputSameDT=on
  "  " : Outport  InitialOutput=0
  wires:
  MinMax1/1 -> MinMax/2
  MAX/1 -> MinMax1/1
  MIN/1 -> MinMax/1
  MinMax/1 -> "  "/1
  In/1 -> MinMax1/2

== system powerlib_extras/Discrete  Control Blocks/Discrete HVDC Controller/Gamma Regulator/Gamma Regulator/Kp Linearisation/S6 ==
  note: Limiter
      | with external
      | limits
  MAX : Inport  Port=1  LatchInput=off
  In : Inport  Port=2  LatchInput=off
  MIN : Inport  Port=3  LatchInput=off
  MinMax : MinMax  Function=max  Inputs=2  SaturateOnIntegerOverflow=on  InputSameDT=on
  MinMax1 : MinMax  Inputs=2  SaturateOnIntegerOverflow=on  InputSameDT=on
  "  " : Outport  InitialOutput=0
  wires:
  MinMax1/1 -> MinMax/2
  MAX/1 -> MinMax1/1
  MIN/1 -> MinMax/1
  MinMax/1 -> "  "/1
  In/1 -> MinMax1/2

== system powerlib_extras/Discrete  Control Blocks/Discrete HVDC Controller/Gamma Regulator/Gamma Regulator/S16/S6 ==
  note: Silvano Casoria
      | Laboratoire simulation de reseaux, IREQ
  note: Limiter
      | with external
      | limits
  MAX : Inport  Port=1  LatchInput=off
  In : Inport  Port=2  LatchInput=off
  MIN : Inport  Port=3  LatchInput=off
  MinMax : MinMax  Function=max  Inputs=2  SaturateOnIntegerOverflow=on  InputSameDT=on
  MinMax1 : MinMax  Inputs=2  SaturateOnIntegerOverflow=on  InputSameDT=on
  "  " : Outport  InitialOutput=0
  wires:
  In/1 -> MinMax1/2
  MinMax/1 -> "  "/1
  MIN/1 -> MinMax/1
  MAX/1 -> MinMax1/1
  MinMax1/1 -> MinMax/2

== system powerlib_extras/Discrete  Control Blocks/Discrete HVDC Controller/Voltage Regulator/Voltage Regulator/Kp Linearisation/S6 ==
  note: Limiter
      | with external
      | limits
  MAX : Inport  Port=1  LatchInput=off
  In : Inport  Port=2  LatchInput=off
  MIN : Inport  Port=3  LatchInput=off
  MinMax : MinMax  Function=max  Inputs=2  SaturateOnIntegerOverflow=on  InputSameDT=on
  MinMax1 : MinMax  Inputs=2  SaturateOnIntegerOverflow=on  InputSameDT=on
  "  " : Outport  InitialOutput=0
  wires:
  In/1 -> MinMax1/2
  MinMax/1 -> "  "/1
  MIN/1 -> MinMax/1
  MAX/1 -> MinMax1/1
  MinMax1/1 -> MinMax/2

== system powerlib_extras/Discrete  Control Blocks/Discrete HVDC Controller/Voltage Regulator/Voltage Regulator/S16/S6 ==
  note: Limiter
      | with external
      | limits
  note: Silvano Casoria
      | Laboratoire simulation de reseaux, IREQ
  MAX : Inport  Port=1  LatchInput=off
  In : Inport  Port=2  LatchInput=off
  MIN : Inport  Port=3  LatchInput=off
  MinMax : MinMax  Function=max  Inputs=2  SaturateOnIntegerOverflow=on  InputSameDT=on
  MinMax1 : MinMax  Inputs=2  SaturateOnIntegerOverflow=on  InputSameDT=on
  "  " : Outport  InitialOutput=0
  wires:
  MinMax1/1 -> MinMax/2
  MAX/1 -> MinMax1/1
  MIN/1 -> MinMax/1
  MinMax/1 -> "  "/1
  In/1 -> MinMax1/2

== system powerlib_extras/Discrete  Control Blocks/Discrete SV PWM Generator/SV Modulator Pattern #1/Generate  pulse pattern/Determine interval of the PWM period based on Ta Tb and To/Subsystem ==
  TaTbTo : Inport  Port=1  LatchInput=off
  "  1/2" : Gain  Gain=0.5  SaturateOnIntegerOverflow=on
  " 1/2" : Gain  Gain=0.5  SaturateOnIntegerOverflow=on
  " 1/2 " : Gain  Gain=0.5  SaturateOnIntegerOverflow=on
  1/4 : Gain  Gain=0.25  SaturateOnIntegerOverflow=on
  Demux : Demux  Outputs=3
  Mux1 : Mux  Inputs=6
  Sum{5..9} (5 alike) : Sum  SaturateOnIntegerOverflow=on
  Timing : Outport
  wires:
  " 1/2 "/1 -> Sum9/2, Sum5/2
  Demux/3 -> " 1/2"/1, 1/4/1
  "  1/2"/1 -> Sum8/2, Sum6/2
  TaTbTo/1 -> Demux/1
  " 1/2"/1 -> Sum7/2
  Demux/2 -> "  1/2"/1
  Demux/1 -> " 1/2 "/1
  1/4/1 -> Sum5/1, Mux1/1
  Sum9/1 -> Mux1/6
  Sum8/1 -> Sum9/1, Mux1/5
  Sum7/1 -> Sum8/1, Mux1/4
  Sum6/1 -> Sum7/1, Mux1/3
  Sum5/1 -> Sum6/1, Mux1/2
  Mux1/1 -> Timing/1
